simulink model "Copter_Plane_F_fs"  (R2020a)
settings: Solver=FixedStepAuto  StartTime=ts  StopTime=ts+700  FixedStep=0.005  RelTol=1e-3
undefined symbols (not defined in the file or in its folder): algo_pitch_in, algo_pwm_out_1, algo_pwm_out_2, algo_pwm_out_3, algo_pwm_out_4, algo_roll_in, algo_throttle_filter, algo_yaw_in, Kd, Ku, Ld, Ldx, Ldy, Lu, Lux, Luy, pwm_max, pwm_min, Qd, QLd, QLdx, QLdy, QLu, QLux, QLuy, Qu, time_algo
settings Model: PauseTimes=600  Creator=a4327  LastModifiedBy=a4327

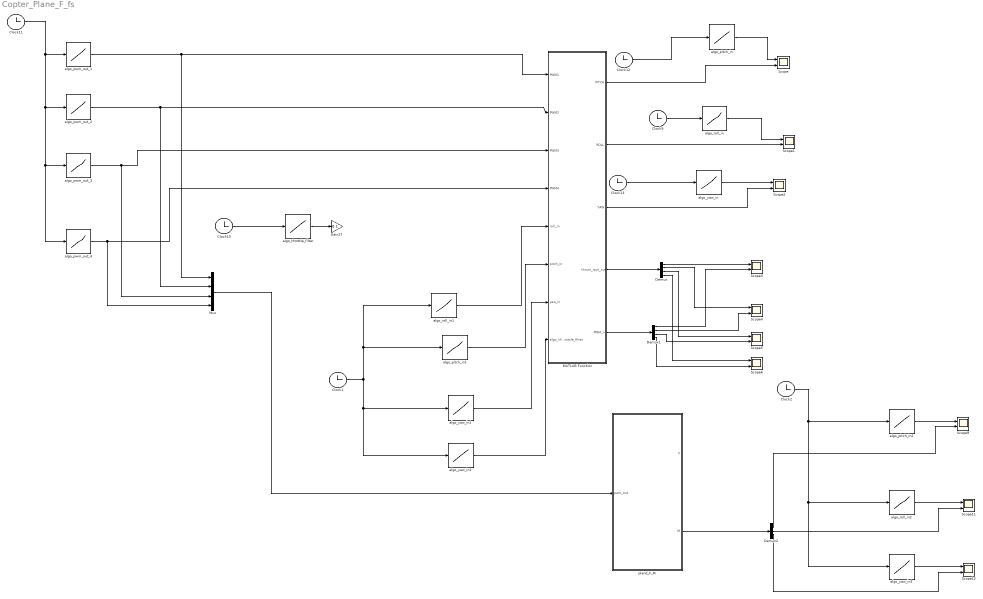
== system Copter_Plane_F_fs ==
  Clock{1..2,9..13} (7 alike) : Clock
  Demux : Demux
  Demux1 : Demux
  Demux2 : Demux  Outputs=3
  Gain27 : Gain  Gain=0.1
  MATLAB Function : MATLAB Function  TreatAsAtomicUnit=on
  Mux : Mux
  Scope{,1..6,9,11..12} (10 alike) : Scope  NumInputPorts=2
  algo_pitch_in : Lookup_n-D  NumberOfTableDimensions=1  BreakpointsForDimension1=time_algo  Table=algo_pitch_in  InternalRulePriority=Speed  RndMeth=Simplest  InputSameDT=on
  algo_pitch_in1 : Lookup_n-D  NumberOfTableDimensions=1  BreakpointsForDimension1=time_algo  Table=algo_pitch_in  InternalRulePriority=Speed  RndMeth=Simplest  InputSameDT=on
  algo_pitch_in2 : Lookup_n-D  NumberOfTableDimensions=1  BreakpointsForDimension1=time_algo  Table=algo_pitch_in  InternalRulePriority=Speed  RndMeth=Simplest  InputSameDT=on
  algo_pwm_out_1 : Lookup_n-D  NumberOfTableDimensions=1  BreakpointsForDimension1=time_algo  Table=algo_pwm_out_1  InternalRulePriority=Speed  RndMeth=Simplest  InputSameDT=on
  algo_pwm_out_2 : Lookup_n-D  NumberOfTableDimensions=1  BreakpointsForDimension1=time_algo  Table=algo_pwm_out_2  InternalRulePriority=Speed  RndMeth=Simplest  InputSameDT=on
  algo_pwm_out_3 : Lookup_n-D  NumberOfTableDimensions=1  BreakpointsForDimension1=time_algo  Table=algo_pwm_out_3  InternalRulePriority=Speed  RndMeth=Simplest  InputSameDT=on
  algo_pwm_out_4 : Lookup_n-D  NumberOfTableDimensions=1  BreakpointsForDimension1=time_algo  Table=algo_pwm_out_4  InternalRulePriority=Speed  RndMeth=Simplest  InputSameDT=on
  algo_roll_in : Lookup_n-D  NumberOfTableDimensions=1  BreakpointsForDimension1=time_algo  Table=algo_roll_in  InternalRulePriority=Speed  RndMeth=Simplest  InputSameDT=on
  algo_roll_in1 : Lookup_n-D  NumberOfTableDimensions=1  BreakpointsForDimension1=time_algo  Table=algo_roll_in  InternalRulePriority=Speed  RndMeth=Simplest  InputSameDT=on
  algo_roll_in2 : Lookup_n-D  NumberOfTableDimensions=1  BreakpointsForDimension1=time_algo  Table=algo_roll_in  InternalRulePriority=Speed  RndMeth=Simplest  InputSameDT=on
  algo_throttle_filter : Lookup_n-D  NumberOfTableDimensions=1  BreakpointsForDimension1=time_algo  Table=algo_throttle_filter  InternalRulePriority=Speed  RndMeth=Simplest  InputSameDT=on
  algo_yaw_in : Lookup_n-D  NumberOfTableDimensions=1  BreakpointsForDimension1=time_algo  Table=algo_yaw_in  InternalRulePriority=Speed  RndMeth=Simplest  InputSameDT=on
  algo_yaw_in1 : Lookup_n-D  NumberOfTableDimensions=1  BreakpointsForDimension1=time_algo  Table=algo_yaw_in  InternalRulePriority=Speed  RndMeth=Simplest  InputSameDT=on
  algo_yaw_in2 : Lookup_n-D  NumberOfTableDimensions=1  BreakpointsForDimension1=time_algo  Table=algo_throttle_filter  InternalRulePriority=Speed  RndMeth=Simplest  InputSameDT=on
  algo_yaw_in3 : Lookup_n-D  NumberOfTableDimensions=1  BreakpointsForDimension1=time_algo  Table=algo_yaw_in  InternalRulePriority=Speed  RndMeth=Simplest  InputSameDT=on
  pland_F_M : MATLAB Function  TreatAsAtomicUnit=on  VariantControl=plane_mode==ENUM_plane_mode.V1000
  wires:
  algo_yaw_in/1 -> Scope2/1
  Clock11/1 -> algo_pwm_out_4/1, algo_pwm_out_3/1, algo_pwm_out_2/1, algo_pwm_out_1/1
  algo_throttle_filter/1 -> Gain27/1
  Clock9/1 -> algo_roll_in/1
  Clock10/1 -> algo_throttle_filter/1
  Clock13/1 -> algo_yaw_in/1
  Clock12/1 -> algo_pitch_in/1
  algo_pwm_out_2/1 -> Mux/2, MATLAB Function/2(PWM2)
  algo_pwm_out_3/1 -> Mux/3, MATLAB Function/3(PWM3)
  algo_pwm_out_4/1 -> Mux/4, MATLAB Function/4(PWM4)
  MATLAB Function/1(PITCH) -> Scope/2
  algo_pitch_in/1 -> Scope/1
  MATLAB Function/2(ROLL) -> Scope1/2
  algo_roll_in/1 -> Scope1/1
  MATLAB Function/3(YAW) -> Scope2/2
  Clock1/1 -> algo_roll_in1/1, algo_pitch_in1/1, algo_yaw_in2/1, algo_yaw_in1/1
  algo_pitch_in1/1 -> MATLAB Function/6(pitch_in)
  algo_yaw_in1/1 -> MATLAB Function/7(yaw_in)
  algo_roll_in1/1 -> MATLAB Function/5(roll_in)
  algo_yaw_in2/1 -> MATLAB Function/8(algo_throttle_filter)
  MATLAB Function/5(PWM_n) -> Demux1/1
  MATLAB Function/4(thrust_rpyt_out) -> Demux/1
  Demux/1 -> Scope3/1
  Demux1/1 -> Scope3/2
  Demux/2 -> Scope4/1
  Demux1/2 -> Scope4/2
  Demux/3 -> Scope5/1
  Demux1/3 -> Scope5/2
  Demux/4 -> Scope6/1
  Demux1/4 -> Scope6/2
  algo_pwm_out_1/1 -> Mux/1, MATLAB Function/1(PWM1)
  Mux/1 -> pland_F_M/1(pwm_out)
  pland_F_M/2(M) -> Demux2/1
  algo_roll_in2/1 -> Scope11/1
  Clock2/1 -> algo_yaw_in3/1, algo_roll_in2/1, algo_pitch_in2/1
  algo_pitch_in2/1 -> Scope9/1
  algo_yaw_in3/1 -> Scope12/1
  Demux2/1 -> Scope9/2
  Demux2/2 -> Scope11/2
  Demux2/3 -> Scope12/2

== matlab function Copter_Plane_F_fs/pland_F_M ==
  settings: updateMethod=DISCRETE
  data: F output; M output; pwm_out input; Ku parameter; Kd parameter; Lux parameter; Luy parameter; Ldx parameter; Ldy parameter; Lu parameter; Ld parameter; pwm_min parameter; pwm_max parameter; Qu parameter; QLux parameter; QLuy parameter; QLu parameter; QLdx parameter; QLdy parameter; QLd parameter; Qd parameter
function [F,M]   = pland_F_M(pwm_out, Ku, Kd, Lux, Luy, Ldx, Ldy, Lu, Ld, pwm_min, pwm_max, Qu, QLux, QLuy, QLu, QLdx, QLdy, QLd, Qd)
    

F1=(pwm_out(1)-pwm_min)/(pwm_max-pwm_min)*Ku;
F2=(pwm_out(2)-pwm_min)/(pwm_max-pwm_min)*Kd;
F3=(pwm_out(3)-pwm_min)/(pwm_max-pwm_min)*Ku;
F4=(pwm_out(4)-pwm_min)/(pwm_max-pwm_min)*Kd;
%  F2=0;
tail_tilt_temp=constrain_value(0,-9000,700);

F24x_g=(F2+F4)*sind(-tail_tilt_temp/100);
F24z_g=(F2+F4)*cosd(-tail_tilt_temp/100);

F_copter=[F24x_g; 0 ;-(F1+F3+F24z_g)];
Mx=(-F1+F3)*Lux+(F2-F4)*Ldx;
% My=(F1+F3)*Luy+(-F2-F4)*Ldy;
My=(F1+F3)*Luy+(-F2-F4)*Ldy*cosd(-tail_tilt_temp/100);
Mz=(-F1+F3)*Lu*sind(Qu)+(-F2+F4)*Ld*sind(Qd);%0.1736=sind(10)  0.1071= Ld*900*sind(10)/(Lu*1600)
Mz_g=(F2-F4)*Ldx*sind(-tail_tilt_temp/100);
% Mz_g=0;
Mz=Mz+Mz_g;
M_copter=[Mx; My; Mz];
%%%%%%%%%%%%%%%%%%%%%%%%%%%%%%%%%%%%%%%%%%%%%%%%%%%%%%%
%% 0 :copter Stabilize,1:copter althold ,2:copter poshold,3:Plane Stabilize 4:Plane TECS; 5：Plane L1

    
    F=F_copter;
    M=M_copter;
%%%%%%%%%%%%%%%%%%%%%%%%%%%%%%%%%%%%%%%%%%%%%%%%%%%%%%%%%%%%
end

== matlab function Copter_Plane_F_fs/MATLAB Function ==
  data: PWM1 input; PITCH output; PWM2 input; PWM3 input; PWM4 input; ROLL output; YAW output; thrust_rpyt_out output; roll_in input; pitch_in input; yaw_in input; PWM_n output; algo_throttle_filter input
function [PITCH,ROLL,YAW,thrust_rpyt_out,PWM_n] = fcn(PWM1, PWM2,PWM3,PWM4,roll_in,pitch_in,yaw_in,algo_throttle_filter)

PITCH = (PWM1+PWM3-PWM2-PWM4)/1000;
ROLL  = (PWM3+PWM2-PWM1-PWM4)/1000;
YAW   = (PWM3+PWM4-PWM1-PWM2)/1000;
PWM_n=([PWM1, PWM2,PWM3,PWM4]-1000)/1000;
roll_factor  =[   -0.7071    0.7071    0.7071   -0.7071];
pitch_factor =[    0.5252   -0.8890    0.5252   -0.8890];
yaw_factor   =[   -1.0000   -2.5599    1.0000    2.5599];
thrust_rpyt_out=[0 0 0 0];
for i=1:4
thrust_rpyt_out(i) = roll_in * roll_factor(i) + pitch_in * pitch_factor(i)+yaw_in*yaw_factor(i)+algo_throttle_filter;
end
PWM_n_o=PWM_n-algo_throttle_filter;
pitch_n=(PWM_n_o(1)+PWM_n_o(3)*-pitch_factor(2)+(PWM_n_o(2)+PWM_n_o(4))*-pitch_factor(1))/(-pitch_factor(1)*pitch_factor(2));
roll_n =((PWM_n_o(2)+PWM_n_o(3))*roll_factor(2)+(PWM_n_o(1)+PWM_n_o(4))*roll_factor(1))/(-roll_factor(1)*roll_factor(2));
yaw_n  =(PWM_n_o(3)*yaw_factor(4)+PWM_n_o(4)*yaw_factor(3)+PWM_n_o(1)*yaw_factor(2)+PWM_n_o(2)*yaw_factor(1))/(yaw_factor(1)*yaw_factor(2));
